simulink model "EV_Charger"  (Simulink 7.0)
settings: Solver=ode23t  StartTime=0.0  StopTime=1.0  RelTol=1e-3
undefined symbols (not defined in the file): Ion, Lithium
libraries: powerlib x21, powerlib_extras x5, simulink x2
settings Model: Creator=Adeboye  LastModifiedBy=Adeboye

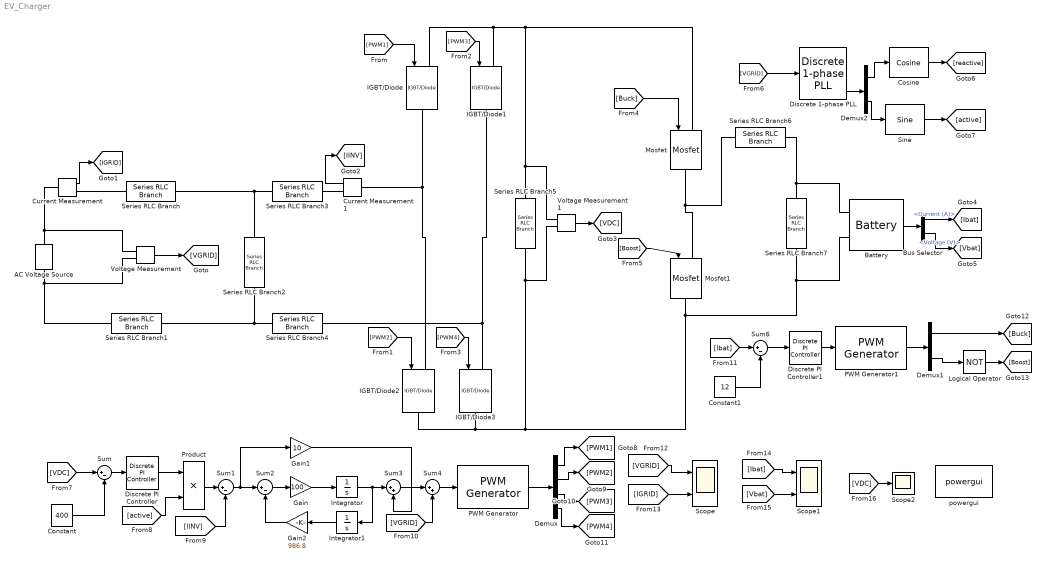
== system EV_Charger ==
  AC Voltage Source : powerlib/Electrical Sources/AC Voltage Source  Orientation=up  DialogController=POWERSYS.PowerSysDialog  SystemSampleTime=-1  Amplitude=325  Phase=0  Frequency=50  SampleTime=0  Measurements=None
  Battery : powerlib/Electrical Sources/Battery  SystemSampleTime=-1  BatType=Lithium-Ion  NomV=160  NomQ=120  SOC=50  ShowDetailedParameters=off  FullV=116  Dis_rate=20  R=0.033333  Normal_OP=98  expZone=[103 85]  Dis_Char=off  current=[1.5 3]  Units=Time
  Bus Selector : BusSelector  OutputSignals=Current (A),Voltage (V)
  Constant : Constant  Value=400  OutDataType=sfix(16)  OutScaling=2^0
  Constant1 : Constant  Value=12  OutDataType=sfix(16)  OutScaling=2^0
  Cosine : simulink/Lookup Tables/Cosine  SystemSampleTime=-1  Formula=cos(2*pi*u)  NumDataPoints=(2^5)+1  OutputWordLength=16
  Current Measurement : powerlib/Measurements/Current Measurement  DialogController=POWERSYS.PowerSysDialog  SystemSampleTime=-1  PhasorSimulation=off  OutputType=Complex  PSBequivalent=0
  Current Measurement1 : powerlib/Measurements/Current Measurement  Orientation=left  DialogController=POWERSYS.PowerSysDialog  SystemSampleTime=-1  PhasorSimulation=off  OutputType=Complex  PSBequivalent=0
  Demux : Demux
  Demux1 : Demux  Outputs=2
  Demux2 : Demux  Outputs=2
  Discrete 1-phase PLL : powerlib_extras/Discrete  Control Blocks/Discrete 1-phase PLL  DialogController=POWERSYS.PowerSysDialog  SystemSampleTime=-1  Fmin=45  Par_Init=[0 50]  ParK=[180 3200]  Ts=1e-6
  Discrete PI Controller : powerlib_extras/Discrete  Control Blocks/Discrete PI Controller  DialogController=POWERSYS.PowerSysDialog  SystemSampleTime=-1  Kp=1  Ki=10  Par_Limits=[1e6 -1e6]  Init=0  Ts=50e-6
  Discrete PI Controller1 : powerlib_extras/Discrete  Control Blocks/Discrete PI Controller  DialogController=POWERSYS.PowerSysDialog  SystemSampleTime=-1  Kp=0.005  Ki=10  Par_Limits=[0.95 0]  Init=0  Ts=50e-6
  Gain : Gain  Gain=100  ParameterDataType=sfix(16)  ParameterScaling=2^0  OutDataType=sfix(16)  OutScaling=2^0
  Gain1 : Gain  Gain=10  ParameterDataType=sfix(16)  ParameterScaling=2^0  OutDataType=sfix(16)  OutScaling=2^0
  Gain2 : Gain  Orientation=left  Gain=986.8  ParameterDataType=sfix(16)  ParameterScaling=2^0  OutDataType=sfix(16)  OutScaling=2^0
  IGBT/Diode{,1..3} (4 alike) : powerlib/Power Electronics/IGBT//Diode  Orientation=down  DialogController=POWERSYS.PowerSysDialog  SystemSampleTime=-1  Ron=1e-3  Rs=1e5  Cs=inf  Measurements=off
  Integrator : Integrator
  Integrator1 : Integrator  Orientation=left
  Logical Operator : Logic  Operator=NOT  AllPortsSameDT=off  OutDataTypeMode=boolean
  Mosfet : powerlib/Power Electronics/Mosfet  Orientation=down  DialogController=POWERSYS.PowerSysDialog  SystemSampleTime=-1  Ron=0.1  Lon=0  Rd=0.01  Vfd=0  IC=0  Rs=1e5  Cs=inf  Measurements=off
  Mosfet1 : powerlib/Power Electronics/Mosfet  Orientation=down  DialogController=POWERSYS.PowerSysDialog  SystemSampleTime=-1  Ron=0.1  Lon=0  Rd=0.01  Vfd=0  IC=0  Rs=1e5  Cs=inf  Measurements=off
  PWM Generator : powerlib_extras/Control  Blocks/PWM Generator  DialogController=POWERSYS.PowerSysDialog  SystemSampleTime=-1  GeneratorMode="2-arm  bridge (4 pulses)"  Fc=10000  Internal=on  mIndex=0.4  Freq=50  Phase=0
  PWM Generator1 : powerlib_extras/Control  Blocks/PWM Generator  DialogController=POWERSYS.PowerSysDialog  SystemSampleTime=-1  GeneratorMode="1-arm  bridge (2 pulses)"  Fc=10000  Internal=on  mIndex=0.4  Freq=50  Phase=0
  Product : Product  OutDataType=sfix(16)  OutScaling=2^0  RndMeth=Zero
  Scope : Scope  NumInputPorts=2
      settings: YMin=-5~-5  YMax=5~5
  Scope1 : Scope  NumInputPorts=2
      settings: YMin=-5~-5  YMax=5~5
  Scope2 : Scope
      settings: SaveName=ScopeData2
  Series RLC Branch : powerlib/Elements/Series RLC Branch  DialogController=POWERSYS.PowerSysDialog  PhysicalDomain=powersysdomain  SubClassName=unknown  LeftPortType=p1  RightPortType=p1  LConnTagsString=__new0  RConnTagsString=__new0  BranchType=L  Resistance=1  Inductance=2.18e-3  SetiL0=off  InitialCurrent=0  Capacitance=1e-6  Setx0=off  InitialVoltage=0  Measurements=None
  Series RLC Branch1 : powerlib/Elements/Series RLC Branch  DialogController=POWERSYS.PowerSysDialog  PhysicalDomain=powersysdomain  SubClassName=unknown  LeftPortType=p1  RightPortType=p1  LConnTagsString=__new0  RConnTagsString=__new0  BranchType=L  Resistance=1  Inductance=2.18e-3  SetiL0=off  InitialCurrent=0  Capacitance=1e-6  Setx0=off  InitialVoltage=0  Measurements=None
  Series RLC Branch2 : powerlib/Elements/Series RLC Branch  Orientation=down  DialogController=POWERSYS.PowerSysDialog  PhysicalDomain=powersysdomain  SubClassName=unknown  LeftPortType=p1  RightPortType=p1  LConnTagsString=__new0  RConnTagsString=__new0  BranchType=C  Resistance=1  Inductance=2.18e-3  SetiL0=off  InitialCurrent=0  Capacitance=6.23e-6  Setx0=off  InitialVoltage=0  Measurements=None
  Series RLC Branch3 : powerlib/Elements/Series RLC Branch  DialogController=POWERSYS.PowerSysDialog  PhysicalDomain=powersysdomain  SubClassName=unknown  LeftPortType=p1  RightPortType=p1  LConnTagsString=__new0  RConnTagsString=__new0  BranchType=L  Resistance=1  Inductance=2.03e-3  SetiL0=off  InitialCurrent=0  Capacitance=1e-6  Setx0=off  InitialVoltage=0  Measurements=None
  Series RLC Branch4 : powerlib/Elements/Series RLC Branch  DialogController=POWERSYS.PowerSysDialog  PhysicalDomain=powersysdomain  SubClassName=unknown  LeftPortType=p1  RightPortType=p1  LConnTagsString=__new0  RConnTagsString=__new0  BranchType=L  Resistance=1  Inductance=2.03e-3  SetiL0=off  InitialCurrent=0  Capacitance=1e-6  Setx0=off  InitialVoltage=0  Measurements=None
  Series RLC Branch5 : powerlib/Elements/Series RLC Branch  Orientation=down  DialogController=POWERSYS.PowerSysDialog  PhysicalDomain=powersysdomain  SubClassName=unknown  LeftPortType=p1  RightPortType=p1  LConnTagsString=__new0  RConnTagsString=__new0  BranchType=RC  Resistance=0.0001  Inductance=1e-3  SetiL0=off  InitialCurrent=0  Capacitance=5600e-6  Setx0=on  InitialVoltage=400  Measurements=None
  Series RLC Branch6 : powerlib/Elements/Series RLC Branch  Orientation=left  DialogController=POWERSYS.PowerSysDialog  PhysicalDomain=powersysdomain  SubClassName=unknown  LeftPortType=p1  RightPortType=p1  LConnTagsString=__new0  RConnTagsString=__new0  BranchType=L  Resistance=0.0001  Inductance=20e-3  SetiL0=off  InitialCurrent=0  Capacitance=5600e-6  Setx0=on  InitialVoltage=400  Measurements=None
  Series RLC Branch7 : powerlib/Elements/Series RLC Branch  Orientation=down  DialogController=POWERSYS.PowerSysDialog  PhysicalDomain=powersysdomain  SubClassName=unknown  LeftPortType=p1  RightPortType=p1  LConnTagsString=__new0  RConnTagsString=__new0  BranchType=RC  Resistance=0.0001  Inductance=20e-3  SetiL0=off  InitialCurrent=0  Capacitance=100e-6  Setx0=off  InitialVoltage=400  Measurements=None
  Sine : simulink/Lookup Tables/Sine  SystemSampleTime=-1  Formula=sin(2*pi*u)  NumDataPoints=(2^5)+1  OutputWordLength=16
  Sum{,1..2,6} (4 alike) : Sum  Inputs=|+-  OutDataType=sfix(16)  OutScaling=2^0
  Sum3 : Sum  Inputs=|++  OutDataType=sfix(16)  OutScaling=2^0
  Sum4 : Sum  Inputs=|++  OutDataType=sfix(16)  OutScaling=2^0
  Voltage Measurement : powerlib/Measurements/Voltage Measurement  DialogController=POWERSYS.PowerSysDialog  SystemSampleTime=-1  PhasorSimulation=off  OutputType=Complex  PSBequivalent=0
  Voltage Measurement1 : powerlib/Measurements/Voltage Measurement  DialogController=POWERSYS.PowerSysDialog  SystemSampleTime=-1  PhasorSimulation=off  OutputType=Complex  PSBequivalent=0
  powergui : powerlib/powergui  SystemSampleTime=-1  SimulationMode=Discrete  SampleTime=1e-6  echomessages=off  RestoreLinks=warning  x0status=blocks  Frange=[0:2:500]  Ylog=off  Xlog=on  ShowGrid=off  save=off  variable=ZData  ZoomFFT=on  StartTime=0.0  cycles=1  DisplayStyle=1  fundamental=60  FreqAxis=off  MaxFrequency=1000  frequencyindice=50  frequencyindicesteady=1  RmsSteady=1  display=off  Ts=0  frequency=60  methode=off  HookPort=off  Interpol=off  SPID=off  FunctionMessages=off
  wires:
  Voltage Measurement/1 -> [VGRID]
  Current Measurement/1 -> [IGRID]
  Current Measurement1/1 -> [IINV]
  [PWM1] -> IGBT/Diode/1
  [PWM2] -> IGBT/Diode2/1
  [PWM3] -> IGBT/Diode1/1
  [PWM4] -> IGBT/Diode3/1
  Voltage Measurement1/1 -> [VDC]
  [Buck] -> Mosfet/1
  [Boost] -> Mosfet1/1
  Battery/1 -> Bus Selector/1
  Bus Selector/1 -> [Ibat]  "<Current (A)>"
  Bus Selector/2 -> [Vbat]  "<Voltage (V)>"
  [VGRID] -> Discrete 1-phase PLL/1
  Cosine/1 -> [reactive]
  Sine/1 -> [active]
  [VDC] -> Sum/1
  Constant/1 -> Sum/2
  Sum/1 -> Discrete PI Controller/1
  Discrete PI Controller/1 -> Product/1
  [active] -> Product/2
  Product/1 -> Sum1/1
  [IINV] -> Sum1/2
  Sum1/1 -> Sum2/1, Gain1/1
  Sum2/1 -> Gain/1
  Gain/1 -> Integrator/1
  Integrator/1 -> Sum3/1, Integrator1/1
  Gain1/1 -> Sum3/2
  Integrator1/1 -> Gain2/1
  Gain2/1 -> Sum2/2
  Sum3/1 -> Sum4/1
  [VGRID] -> Sum4/2
  Sum4/1 -> PWM Generator/1
  PWM Generator/1 -> Demux/1
  Demux/1 -> [PWM1]
  Demux/2 -> [PWM2]
  Demux/3 -> [PWM3]
  Demux/4 -> [PWM4]
  [Ibat] -> Sum6/1
  Constant1/1 -> Sum6/2
  Sum6/1 -> Discrete PI Controller1/1
  Logical Operator/1 -> [Boost]
  [VGRID] -> Scope/1
  [IGRID] -> Scope/2
  [Ibat] -> Scope1/1
  [Vbat] -> Scope1/2
  [VDC] -> Scope2/1
  Discrete PI Controller1/1 -> PWM Generator1/1
  PWM Generator1/1 -> Demux1/1
  Demux1/1 -> [Buck]
  Demux1/2 -> Logical Operator/1
  Discrete 1-phase PLL/3 -> Demux2/1
  Demux2/1 -> Cosine/1
  Demux2/2 -> Sine/1
  connections:
  AC Voltage Source/RConn1 -- Current Measurement/LConn1 -- Voltage Measurement/LConn1
  Series RLC Branch1/LConn1 -- Voltage Measurement/LConn2 -- AC Voltage Source/LConn1
  Series RLC Branch3/LConn1 -- Series RLC Branch/RConn1 -- Series RLC Branch2/LConn1
  Series RLC Branch4/LConn1 -- Series RLC Branch2/RConn1 -- Series RLC Branch1/RConn1
  Current Measurement1/RConn1 -- Series RLC Branch3/RConn1
  Current Measurement/RConn1 -- Series RLC Branch/LConn1
  IGBT/Diode/RConn1 -- IGBT/Diode2/LConn1 -- Current Measurement1/LConn1
  IGBT/Diode1/RConn1 -- IGBT/Diode3/LConn1 -- Series RLC Branch4/RConn1
  Series RLC Branch7/RConn1 -- Mosfet1/RConn1 -- Series RLC Branch5/RConn1 -- Voltage Measurement1/LConn2 -- IGBT/Diode2/RConn1 -- IGBT/Diode3/RConn1 -- Battery/LConn2
  IGBT/Diode1/LConn1 -- IGBT/Diode/LConn1 -- Series RLC Branch5/LConn1 -- Voltage Measurement1/LConn1 -- Mosfet/LConn1
  Mosfet/RConn1 -- Mosfet1/LConn1 -- Series RLC Branch6/RConn1
  Series RLC Branch6/LConn1 -- Series RLC Branch7/LConn1 -- Battery/LConn1
